simulink model "firinterpolation_ref2"  (Simulink 4.00)
settings: Solver=FixedStepDiscrete  StartTime=0.0  StopTime=30  RelTol=1e-3
PreLoadFcn:
  | load mtlb; whos mtlb Fs
PostLoadFcn:
  | set_param(gcs,'SimulationCommand','Update')
libraries: dspmlti3 x1, dspsrcs3 x1
settings Model: RequirementInfo=9  LastModifiedBy=dfass  LimitDataPoints=off  ExtModeTrigMode=oneshot  ExtModeArmWhenConnect=off  BlockReductionOpt=off

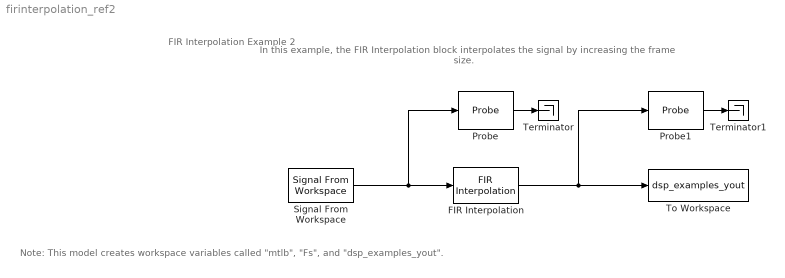
== system firinterpolation_ref2 ==
  note: FIR Interpolation Example 2
  note: In this example, the FIR Interpolation block interpolates the
      | signal by increasing the frame size.
  note: Note: This model creates workspace variables called "mtlb", "Fs", and "dsp_examples_yout".
  FIR Interpolation : dspmlti3/FIR Interpolation  h=fir1(15,1/4)  L=4  framing=Maintain input frame rate
  Probe : Probe  ProbeWidth=off  ProbeSampleTime=on  ProbeComplexSignal=off  ProbeSignalDimensions=off
  Probe1 : Probe  ProbeWidth=off  ProbeSampleTime=on  ProbeComplexSignal=off  ProbeSignalDimensions=off
  Signal From Workspace : dspsrcs3/Signal From Workspace  X=mtlb  Ts=1/16  nsamps=16  OutputAfterFinalValue=Setting To Zero
  Terminator : Terminator
  Terminator1 : Terminator
  To Workspace : ToWorkspace  VariableName=dsp_examples_yout  SampleTime=-1  SaveFormat=Array
  wires:
  FIR Interpolation/1 -> To Workspace/1, Probe1/1
  Signal From Workspace/1 -> Probe/1, FIR Interpolation/1
  Probe/1 -> Terminator/1
  Probe1/1 -> Terminator1/1
